simulink model "follower_v3"  (R2024a)
settings: Solver=VariableStepAuto  StartTime=0.0  StopTime=inf  RelTol=1e-3
undefined symbols (not defined in the file): linear
libraries: ros2lib x4
settings Model: Creator=eswarm  LastModifiedBy=eswarm

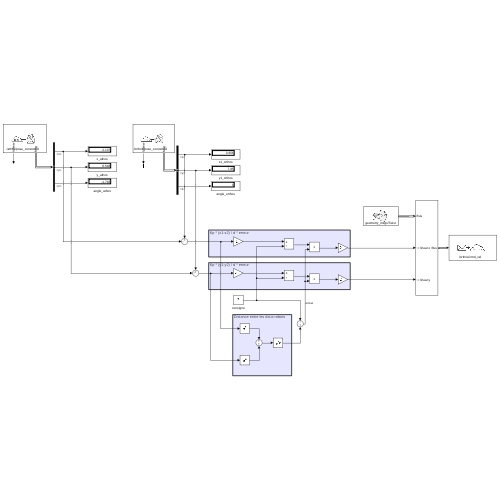
[thumbnail: Simulink's stored preview of the top-level diagram]
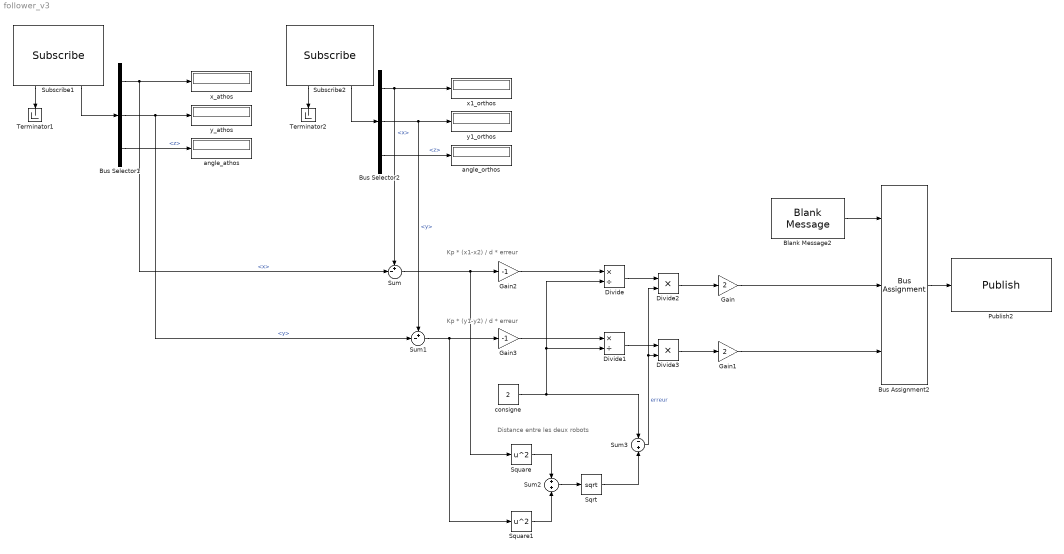
== system follower_v3 ==
  note: Kp * (x1-x2) / d * erreur
  note: Distance entre les deux robots
  note: Kp * (y1-y2) / d * erreur
  Blank Message2 : ros2lib/Blank Message  messageClass=Message  entityType=geometry_msgs/Twist  messageType=geometry_msgs/Twist  SampleTime=0.1
  Bus Assignment2 : BusAssignment  AssignedSignals=linear.x,linear.y
  Bus Selector1 : BusSelector  OutputSignals=position.x,position.y,orientation.z
  Bus Selector2 : BusSelector  OutputSignals=position.x,position.y,orientation.z
  Divide : Product  Inputs=*/  RndMeth=Zero  SaturateOnIntegerOverflow=on
  Divide1 : Product  Inputs=*/  RndMeth=Zero  SaturateOnIntegerOverflow=on
  Divide2 : Product  Inputs=**  RndMeth=Zero  SaturateOnIntegerOverflow=on
  Divide3 : Product  Inputs=**  RndMeth=Zero  SaturateOnIntegerOverflow=on
  Gain : Gain  Gain=2
  Gain1 : Gain  Gain=2
  Gain2 : Gain  Gain=-1
  Gain3 : Gain  Gain=-1
  Publish2 : ros2lib/Publish  topicSource=Select from ROS network  topic=/orthos/cmd_vel  messageType=geometry_msgs/Twist  QOSHistory=Keep last  QOSDepth=1  QOSReliability=Reliable  QOSDurability=Volatile  QOSDeadline=Inf  QOSLifespan=Inf  QOSLiveliness=Automatic  QOSLeaseDuration=Inf  QOSAvoidROSNamespaceConventions=off
  Sqrt : Sqrt
  Square : Math  Operator=square
  Square1 : Math  Operator=square
  Subscribe1 : ros2lib/Subscribe  topicSource=Select from ROS network  topic=/athos/pose_converted  messageType=geometry_msgs/Pose  sampleTime=0.1  QOSHistory=Keep last  QOSDepth=1  QOSReliability=Reliable  QOSDurability=Volatile  QOSDeadline=Inf  QOSLifespan=Inf  QOSLiveliness=Automatic  QOSLeaseDuration=Inf  QOSAvoidROSNamespaceConventions=off
  Subscribe2 : ros2lib/Subscribe  topicSource=Select from ROS network  topic=/orthos/pose_converted  messageType=geometry_msgs/Pose  sampleTime=0.1  QOSHistory=Keep last  QOSDepth=1  QOSReliability=Reliable  QOSDurability=Volatile  QOSDeadline=Inf  QOSLifespan=Inf  QOSLiveliness=Automatic  QOSLeaseDuration=Inf  QOSAvoidROSNamespaceConventions=off
  Sum : Sum  Inputs=+-|
  Sum1 : Sum  Inputs=+-|
  Sum2 : Sum  Inputs=+|+
  Sum3 : Sum  Inputs=-|+
  Terminator1 : Terminator
  Terminator2 : Terminator
  angle_athos : Display
  angle_orthos : Display
  consigne : Constant  Value=2
  x1_orthos : Display
  x_athos : Display
  y1_orthos : Display
  y_athos : Display
  wires:
  Subscribe1/2 -> Bus Selector1/1
  Subscribe1/1 -> Terminator1/1
  Bus Selector1/1 -> Sum/2, x_athos/1  "<x>"
  Bus Selector1/2 -> Sum1/2, y_athos/1  "<y>"
  Bus Selector1/3 -> angle_athos/1  "<z>"
  Bus Selector2/1 -> x1_orthos/1, Sum/1  "<x>"
  Subscribe2/2 -> Bus Selector2/1
  Bus Selector2/3 -> angle_orthos/1  "<z>"
  Subscribe2/1 -> Terminator2/1
  Bus Selector2/2 -> Sum1/1, y1_orthos/1  "<y>"
  Bus Assignment2/1 -> Publish2/1
  Blank Message2/1 -> Bus Assignment2/1
  Gain/1 -> Bus Assignment2/2
  Gain1/1 -> Bus Assignment2/3
  Sum1/1 -> Square1/1, Gain3/1
  Sum/1 -> Gain2/1, Square/1
  Square/1 -> Sum2/1
  Square1/1 -> Sum2/2
  Sum2/1 -> Sqrt/1
  consigne/1 -> Divide1/2, Divide/2, Sum3/1
  Sqrt/1 -> Sum3/2
  Gain2/1 -> Divide/1
  Gain3/1 -> Divide1/1
  Divide/1 -> Divide2/1
  Divide1/1 -> Divide3/1
  Sum3/1 -> Divide2/2, Divide3/2  "erreur"
  Divide2/1 -> Gain/1
  Divide3/1 -> Gain1/1
